simulink model "model"  (R2013b)
settings: Solver=ode45  SolverMode=SingleTasking  StartTime=0.0  StopTime=30  RelTol=1e-3
undefined symbols (not defined in the file): B, F, G, M, V1, W, Y
settings Model: CovMetricSettings=dwe  CovHtmlReporting=off  covSaveCumulativeToWorkspaceVar=off  CovSaveSingleToWorkspaceVar=off  CovExternalEMLEnable=on  Creator=ali  LastModifiedBy=ali
settings DataIOCC: LimitDataPoints=off  SaveFormat=StructureWithTime  ReturnWorkspaceOutputs=on
settings DebuggingCC: UnderspecifiedInitializationDetection=Simplified  MergeDetectMultiDrivingBlocksExec=error  SolverPrmCheckMsg=none  FrameProcessingCompatibilityMsg=error  SFUnexpectedBacktrackingDiag=error  SFNoUnconditionalDefaultTransitionDiag=error
settings HardwareCC: ProdBitPerPointer=64  ProdLargestAtomicFloat=Float  ProdIntDivRoundTo=Zero  ProdEndianess=LittleEndian  ProdHWDeviceType=Specified
settings ModelReferenceCC: PropagateSignalLabelsOutOfModel=on
settings SFSimCC: SimUseLocalCustomCode=on
settings RTWCC: RTWUseLocalCustomCode=on
settings GRTTargetCC: CodeReplacementLibrary=C99 (ISO)  GeneratePreprocessorConditionals=Use local settings

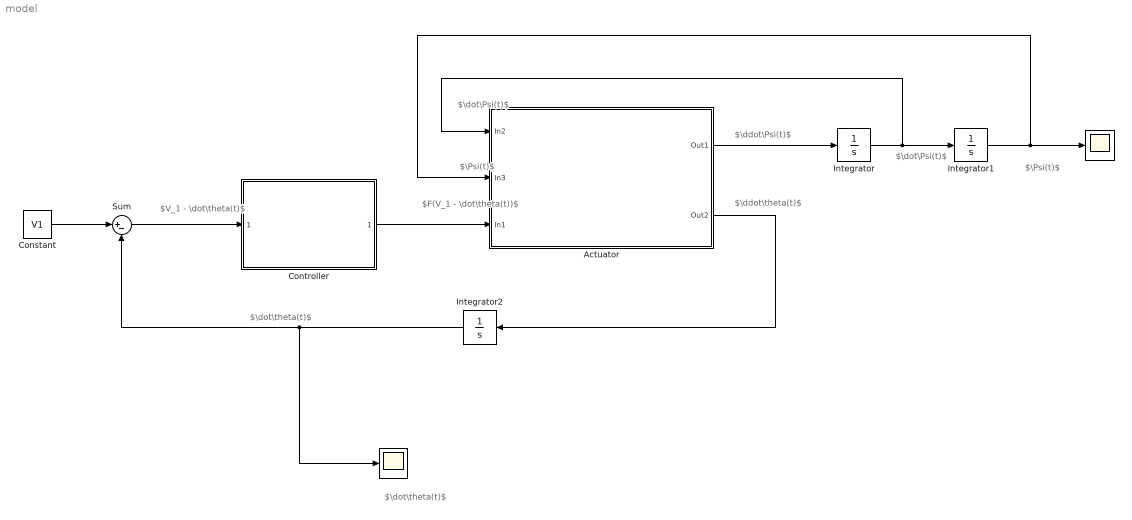
== system model ==
  note: $\ddot\Psi(t)$
  note: $\Psi(t)$
  note: $V_1 - \dot\theta(t)$
  note: $F(V_1 - \dot\theta(t))$
  note: $\Psi(t)$
  note: $\dot\Psi(t)$
  note: $\dot\Psi(t)$
  note: $\ddot\theta(t)$
  note: $\dot\theta(t)$
  note: $\dot\theta(t)$
  " " : Scope
      settings: TimeRange=auto  MaxDataPoints=5000  SaveToWorkspace=off  SaveName=ScopeData  YMin=-10  YMax=10  SampleTime=-1
  " " : Scope
      settings: TimeRange=auto  MaxDataPoints=5000  SaveToWorkspace=off  YMin=-1.27437  YMax=14.93539  SampleTime=-1
  "Actuator " : Subsystem
  Constant : Constant  Value=V1
  Controller : Subsystem
  Integrator : Integrator
  Integrator1 : Integrator
  Integrator2 : Integrator
  Sum : Sum  Inputs=|+-
  wires:
  Sum/1 -> Controller/1(" ")
  Constant/1 -> Sum/1
  Integrator/1 -> "Actuator "/1(In2), Integrator1/1
  Integrator1/1 -> "Actuator "/2(In3), " "/1
  Controller/1(" ") -> "Actuator "/3(In1)
  "Actuator "/1(Out1) -> Integrator/1
  "Actuator "/2(Out2) -> Integrator2/1
  Integrator2/1 -> " "/1, Sum/2

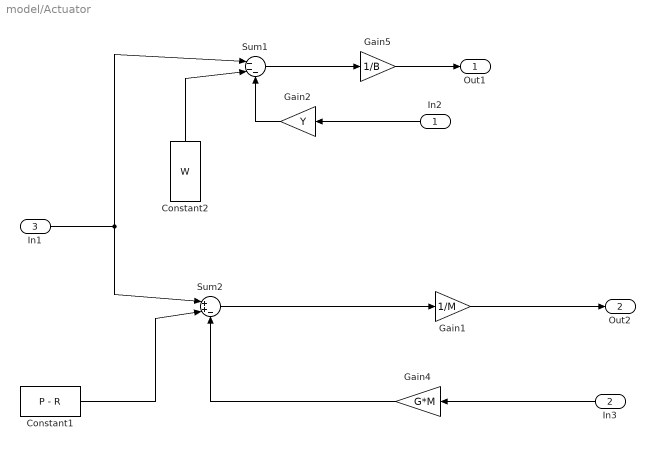
== system model/Actuator  ==
  In2 : Inport
  In3 : Inport  Port=2
  In1 : Inport  Port=3
  Constant1 : Constant  Value=P - R
  Constant2 : Constant  Value=W
  Gain1 : Gain  Gain=1/M
  Gain2 : Gain  Gain=Y
  Gain4 : Gain  Gain=G*M
  Gain5 : Gain  Gain=1/B
  Sum1 : Sum  Inputs=|---
  Sum2 : Sum  Inputs=|++-
  Out1 : Outport
  Out2 : Outport  Port=2
  wires:
  Gain2/1 -> Sum1/3
  In3/1 -> Gain4/1
  In1/1 -> Sum2/1, Sum1/1
  Sum2/1 -> Gain1/1
  In2/1 -> Gain2/1
  Gain5/1 -> Out1/1
  Gain4/1 -> Sum2/3
  Constant2/1 -> Sum1/2
  Gain1/1 -> Out2/1
  Sum1/1 -> Gain5/1
  Constant1/1 -> Sum2/2

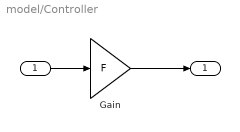
== system model/Controller ==
  " " : Inport
  Gain : Gain  Gain=F
  " " : Outport
  wires:
  Gain/1 -> " "/1
  " "/1 -> Gain/1
